simulink model "Hover_ITAE_sub"  (Simulink 6.6)
settings: Solver=ode45  StartTime=0.0  StopTime=10.0  RelTol=1e-3
libraries: simulink_extras x3
settings Model: Creator=user  LastModifiedBy=user

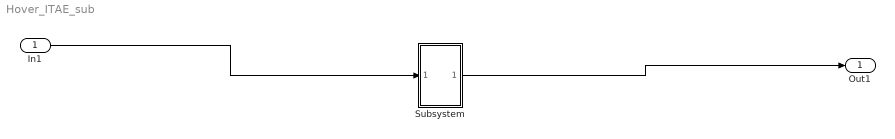
== system Hover_ITAE_sub ==
  In1 : Inport
  Subsystem : Subsystem
  Out1 : Outport
  wires:
  In1/1 -> Subsystem/1(In1)
  Subsystem/1(Out1) -> Out1/1

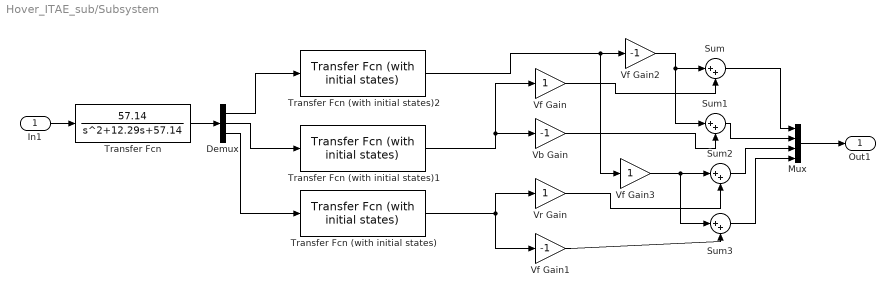
== system Hover_ITAE_sub/Subsystem ==
  In1 : Inport
  Demux : Demux  Outputs=3
  Mux : Mux
  Sum{,1..3} (4 alike) : Sum  Inputs=|++
  Transfer Fcn : TransferFcn  Numerator=[57.14]  Denominator="[1  12.29 57.14]"
  Transfer Fcn (with initial states) : simulink_extras/Additional Linear/Transfer Fcn (with initial states)  SystemSampleTime=-1  N=[20.65 253.7 1180]  D=[1 0]  X0=0
  Transfer Fcn (with initial states)1 : simulink_extras/Additional Linear/Transfer Fcn (with initial states)  SystemSampleTime=-1  N=[20.65 253.7 1180]  D=[1 0]  X0=0
  Transfer Fcn (with initial states)2 : simulink_extras/Additional Linear/Transfer Fcn (with initial states)  SystemSampleTime=-1  N=[134.2 1649 7669]  D=[1 0]  X0=0
  Vb Gain : Gain  Gain=-1
  Vf Gain : Gain
  Vf Gain1 : Gain  Gain=-1
  Vf Gain2 : Gain  Gain=-1
  Vf Gain3 : Gain
  Vr Gain : Gain
  Out1 : Outport
  wires:
  Demux/2 -> Transfer Fcn (with initial states)1/1
  Demux/3 -> Transfer Fcn (with initial states)/1
  Transfer Fcn (with initial states)1/1 -> Vf Gain/1, Vb Gain/1
  Transfer Fcn (with initial states)/1 -> Vr Gain/1, Vf Gain1/1
  Transfer Fcn (with initial states)2/1 -> Vf Gain2/1, Vf Gain3/1
  Vf Gain2/1 -> Sum/1, Sum1/1
  Vf Gain/1 -> Sum/2
  Vb Gain/1 -> Sum1/2
  Vf Gain3/1 -> Sum2/1, Sum3/1
  Vr Gain/1 -> Sum2/2
  Vf Gain1/1 -> Sum3/2
  Sum/1 -> Mux/1
  Sum1/1 -> Mux/2
  Sum2/1 -> Mux/3
  Mux/1 -> Out1/1
  Sum3/1 -> Mux/4
  Transfer Fcn/1 -> Demux/1
  In1/1 -> Transfer Fcn/1
  Demux/1 -> Transfer Fcn (with initial states)2/1
